simulink model "sysgenStreamedFFT"  (Simulink 7.4)
settings: Solver=VariableStepDiscrete  StartTime=0.0  StopTime=3000  RelTol=1e-3
values from neighbouring files (symbols this model uses):
  blue = blue(1:(min_x*min_y))    [makematrix.m]    (also in rgb.mat = [0 0 0 255 255 255 255 255 255 0 0 0 ... (256 elements, 256x)
  c = c(:)    [cellpipe_r13.m]    (also in cordic_sincos_script.m = xSignal; get_pipestr_r13.m = cellpipe_r13(pipestr))
  comp = [zeros(70,2) [zeros(2,66); comp; zeros(2,66)] zeros(70,2)]    [sysgenDWT_StopFcn.m]
undefined symbols (not defined in the file or in its folder): gcbh, xlBlockLoadCallback, xlipgetpartsetting
libraries: xbsIndex_r4 x117, dspxfrm3 x2, xbsCopyrightNotice_r4 x1
(part 1 of 3)
settings Model: Creator=douangp  LastModifiedBy=douangp
settings OptimizationCC: InitFltsAndDblsToZero=on
settings DebuggingCC: SaveWithParameterizedLinksMsg=none  SignalResolutionControl=TryResolveAllWithWarning  MultiTaskDSMMsg=warning  MultiTaskCondExecSysMsg=none
settings RTWCC: IncludeERTFirstTime=on
settings GRTTargetCC: TargetFcnLib=ansi_tfl_tmw.mat

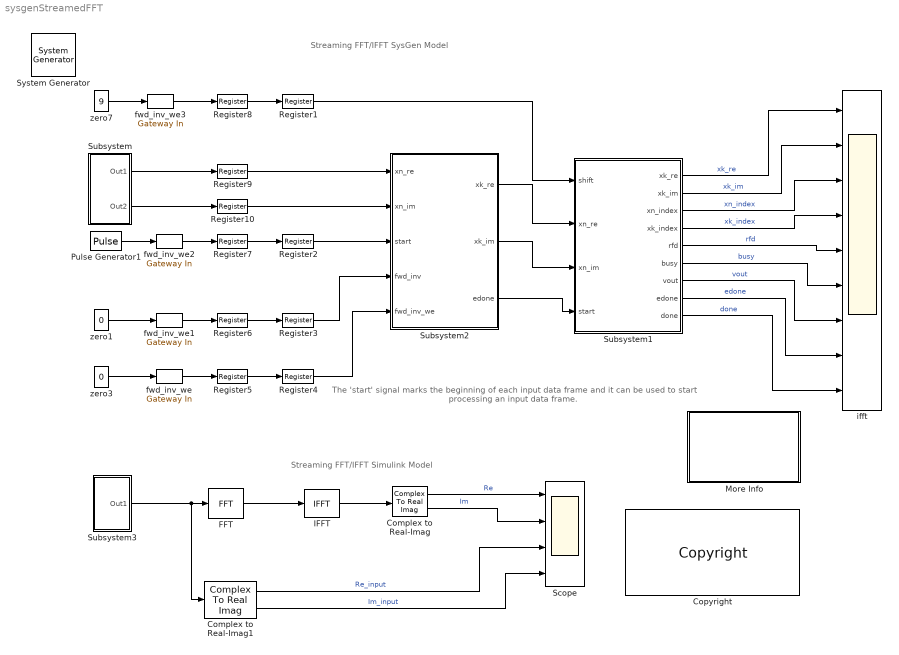
== system sysgenStreamedFFT ==
  note: The 'start' signal marks the beginning of each input data
      | frame and it can be used to start processing an input data frame.
  note: Streaming FFT/IFFT Simulink Model
  note: Streaming FFT/IFFT SysGen Model
  " System Generator" : xbsIndex_r4/ System Generator  Tag=genX  SystemSampleTime=-1  xilinxfamily=virtex6  part=xc6vlx240t  speed=-1  package=ff1156  synthesis_tool=XST  clock_wrapper=Clock Enables  directory=./timing  testbench=off  simulink_period=1  sysclk_period=5  dcm_input_clock_period=100  incr_netlist=off  trim_vbits=Everywhere in SubSystem  dbl_ovrd=According to Block Masks  core_generation=According to Block Masks  run_coregen=off  deprecated_control=off  eval_field=0  block_type=sysgen
      settings: block_version=9.1
  Complex to Real-Imag : ComplexToRealImag
  Complex to Real-Imag1 : ComplexToRealImag
  Copyright : xbsCopyrightNotice_r4/Copyright  copyrighttext="Copyright (c) 2010  by  Xilinx, Inc. All rights reserved.<br><br>This file contains proprietary, confidential information of Xilinx, Inc., is distributed under licensefrom Xilinx, Inc., and may be used, copied and/or disclosed only pursuant to the terms of a valid licenseagreement with Xilinx, Inc. Xilinx hereby grants you a license to use this file solely for design,simulation, implementation and creation of design files limited to Xilinx devices or technologies. Use with non-Xilinx devices or technologies is expressly prohibited and immediately terminates your license unless covered by a separate agreement.<br><br>Xilinx is providing this design, code, or information \"as-is\" solely for use in developing programs and solutions for Xilinx devices, with no obligation on the part of Xilinx to provide support. By providingthis design, code, or information as one possible implementation of this feature, application or standard,Xilinx is making no representation that this implementation is free from any claims of infringement. Youare responsible for obtaining any rights you may require for your implementation. Xilinx expressly disclaimsany warranty whatsoever with respect to the adequacy of the implementation, including but not limited to anywarranties or representations that this implementation is free from claims of infringement, implied warrantiesof merchantability or fitness for a particular purpose.<br><br>Xilinx products are not intended for use in life support appliances, devices, or systems. Use in such applications is expressly prohibited.<br><br>Any modifications that are made to the Source Code are done at the user's sole risk and will be unsupported.<br><br>This copyright and support notice must be retained as part of this text at all times. (c) Copyright 1995-2010 Xilinx, Inc. All rights reserved."  block_type=copyright
      settings: block_version=10.1.00
      settings: infoedit=|
      | Copyright(C) 2008 by  Xilinx, Inc. All rights reserved.<br>
      | <br>
      | This file contains proprietary, confidential information of Xilinx, Inc., is distributed under license
      | from Xilinx, Inc., and may be used, copied and/or disclosed only pursuant to the terms of a valid license
      | agreement with Xilinx, Inc. Xilinx hereby grants you a license to use this file solely for design,
      | simulation, implementation and creation of design files limited to Xilinx devices or technologies. Use
      | with non-Xilinx devices or technologies is expressly prohibited and immediately terminates your license
      | unless covered by a separate agreement.<br>
      | <br>
      | Xilinx is providing this design, code, or information "as-is" solely for use in developing programs and
      | solutions for Xilinx devices, with no obligation on the part of Xilinx to provide support. By providing
      | this design, code, or information as one possible implementation of this feature, application or standard,
      | Xilinx is making no representation that this implementation is free from any claims of infringement. You
      | are responsible for obtaining any rights you may require for your implementation. Xilinx expressly disclaims
      | any warranty whatsoever with respect to the adequacy of the implementation, including but not limited to any
      | warranties or representations that this implementation is free from claims of infringement, implied warranties
      | of merchantability or fitness for a particular purpose.<br>
      | <br>
      | Xilinx products are not intended for use in life support appliances, devices, or systems. Use in such
      | applications is expressly prohibited.<br>
      | <br>
      | Any modifications that are made to the Source Code are done at the user's sole risk and will be unsupported.<br>
      | <br>
      | This copyright and support notice must be retained as part of this text at all times.
      | (c) Copyright 1995-2008 Xilinx, Inc. All rights reserved.
  FFT : dspxfrm3/FFT  DialogController=dspDDGCreate  DialogControllerArgs=DataTag1  CompMethod=Table lookup  TableOpt=HYBRID  TableOptActive=Speed  BitRevOrder=off  InheritFFTLength=on  FFTLength=64  SkipNorm=off  roundingMode=Floor  overflowMode=off
  IFFT : dspxfrm3/IFFT  DialogController=dspDDGCreate  DialogControllerArgs=DataTag2  CompMethod=Table lookup  TableOpt=HYBRID  TableOptActive=Speed  BitRevOrder=off  cs_in=off  SkipNorm=on  InheritFFTLength=on  FFTLength=64  mode=Complex  outSamplingMode=Frame based  roundingMode=Floor  overflowMode=off
  More Info : Subsystem
      mask Display: disp('Double click\n for\n more information.')
  Pulse Generator1 : DiscretePulseGenerator  Amplitude=1  Period=10000  PulseWidth=9999  PhaseDelay=2  SampleTime=1
  Register{1..10} (10 alike) : xbsIndex_r4/Register  init=0  rst=off  en=off  dbl_ovrd=off  block_type=register
      settings: block_version=9.1
  Scope : Scope  NumInputPorts=4
      settings: TimeRange=100  YMin=5.55112e-017~-1~5.55112e-017~-1  YMax=1~1~1~1  SaveName=ScopeData3
  Subsystem : Subsystem
  Subsystem1 : Subsystem
  Subsystem2 : Subsystem
  Subsystem3 : Subsystem
  fwd_inv_we : xbsIndex_r4/Gateway In  arith_type=Boolean  n_bits=16  bin_pt=0  quantization=Truncate  overflow=Wrap  period=1  dbl_ovrd=off  timing_constraint=None  locs_specified=off  LOCs={}  hdl_port=on  block_type=gatewayin
      settings: infoedit="Gateway in block.  Converts inputs of type Simulink integer, double and fixed point to  Xilinx fixed point type.<P><P>Hardware notes:  In hardware these blocks become top level input ports."  xl_area=[0, 0, 0, 0, 0, 0, 0]  block_version=8.2.02
  fwd_inv_we1 : xbsIndex_r4/Gateway In  arith_type=Boolean  n_bits=16  bin_pt=0  quantization=Truncate  overflow=Wrap  period=1  dbl_ovrd=off  timing_constraint=None  locs_specified=off  LOCs={}  hdl_port=on  block_type=gatewayin
      settings: infoedit="Gateway in block.  Converts inputs of type Simulink integer, double and fixed point to  Xilinx fixed point type.<P><P>Hardware notes:  In hardware these blocks become top level input ports."  xl_area=[0, 0, 0, 0, 0, 0, 0]  block_version=8.2.02
  fwd_inv_we2 : xbsIndex_r4/Gateway In  arith_type=Boolean  n_bits=16  bin_pt=0  quantization=Truncate  overflow=Wrap  period=1  dbl_ovrd=off  timing_constraint=None  locs_specified=off  LOCs={}  hdl_port=on  block_type=gatewayin
      settings: infoedit="Gateway in block.  Converts inputs of type Simulink integer, double and fixed point to  Xilinx fixed point type.<P><P>Hardware notes:  In hardware these blocks become top level input ports."  xl_area=[0, 0, 0, 0, 0, 0, 0]  block_version=8.2.02
  fwd_inv_we3 : xbsIndex_r4/Gateway In  arith_type=Unsigned  n_bits=4  bin_pt=0  quantization=Truncate  overflow=Wrap  period=1  dbl_ovrd=off  timing_constraint=None  locs_specified=off  LOCs={}  hdl_port=on  block_type=gatewayin
      settings: infoedit="Gateway in block.  Converts inputs of type Simulink integer, double and fixed point to  Xilinx fixed point type.<P><P>Hardware notes:  In hardware these blocks become top level input ports."  xl_area=[0, 0, 0, 0, 0, 0, 0]  block_version=8.2.02
  ifft : Scope  NumInputPorts=9
      settings: TimeRange=1000  YMin=-0.15~-0.15~0~0~0.95~0.95~0~0~0  YMax=0.15~0.15~300~300~1.05~1.05~1~1~1
  zero1 : Constant  Value=0  OutDataType=sfix(16)  OutScaling=2^0
  zero3 : Constant  Value=0  OutDataType=sfix(16)  OutScaling=2^0
  zero7 : Constant  Value=9  OutDataType=sfix(16)  OutScaling=2^0
  wires:
  Register10/1 -> Subsystem2/2(xn_im)
  Register4/1 -> Subsystem2/5(fwd_inv_we)
  fwd_inv_we/1 -> Register5/1
  zero3/1 -> fwd_inv_we/1
  Subsystem1/1(xk_re) -> ifft/1  "xk_re"
  Subsystem1/2(xk_im) -> ifft/2  "xk_im"
  Subsystem1/3(xn_index) -> ifft/3  "xn_index"
  Subsystem1/4(xk_index) -> ifft/4  "xk_index"
  Subsystem1/5(rfd) -> ifft/5  "rfd"
  Subsystem1/6(busy) -> ifft/6  "busy"
  Subsystem1/7(vout) -> ifft/7  "vout"
  Subsystem1/8(edone) -> ifft/8  "edone"
  Subsystem1/9(done) -> ifft/9  "done"
  Subsystem/2(Out2) -> Register10/1
  Subsystem/1(Out1) -> Register9/1
  Register5/1 -> Register4/1
  FFT/1 -> IFFT/1
  IFFT/1 -> Complex to Real-Imag/1
  Complex to Real-Imag/1 -> Scope/1  "Re"
  Complex to Real-Imag/2 -> Scope/2  "Im"
  Complex to Real-Imag1/2 -> Scope/4  "Im_input"
  Complex to Real-Imag1/1 -> Scope/3  "Re_input"
  Register9/1 -> Subsystem2/1(xn_re)
  Subsystem2/1(xk_re) -> Subsystem1/2(xn_re)
  Subsystem2/2(xk_im) -> Subsystem1/3(xn_im)
  Subsystem2/3(edone) -> Subsystem1/4(start)
  Subsystem3/1(Out1) -> FFT/1, Complex to Real-Imag1/1
  fwd_inv_we3/1 -> Register8/1
  zero7/1 -> fwd_inv_we3/1
  Register1/1 -> Subsystem1/1(shift)
  fwd_inv_we1/1 -> Register6/1
  Register6/1 -> Register3/1
  Register3/1 -> Subsystem2/4(fwd_inv)
  zero1/1 -> fwd_inv_we1/1
  fwd_inv_we2/1 -> Register7/1
  Register7/1 -> Register2/1
  Register2/1 -> Subsystem2/3(start)
  Register8/1 -> Register1/1
  Pulse Generator1/1 -> fwd_inv_we2/1

== system sysgenStreamedFFT/More Info ==
  note: This design demonstrates how the Xilinx FFT block can be used in a data stream with identical input and output rates.
      | In addition, the demo also shows how to incorporate DDS Compiler blocks and complex multipliers as a subsystem to this model.
      | Both Sine and Cosine output signals are used as inputs into the complex multipliers, realized and verified using Simulink, fixed-point simulation.
      | A Simulink model is provided for your reference only.
      |
      | Using SysGen and ISE 10.1, the following operating frequency is obtained for these two target devices:
      | -  Virtex-5 xc5vsx50t-1ff1136:  3.236 ns with 5 levels of logic
      | -  Spartan-3A DSP xc3sd3400a-4fg676: 5.655 ns with 7 levels of logic
  note: Streaming FFT/IFFT Demonstration

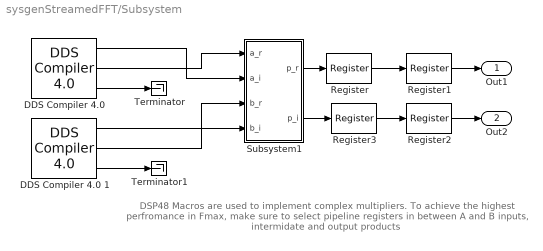
== system sysgenStreamedFFT/Subsystem ==
  note: DSP48 Macros are used to implement complex multipliers. To achieve
      | the highest perfromance in Fmax, make sure to select pipeline registers in between
      | A and B inputs, intermidate and output products
  "DDS Compiler 4.0 " : xbsIndex_r4/DDS Compiler 4.0   partspresent=Phase_Generator_and_SIN_COS_LUT  dds_clock_rate=100  channels=1  parameter_entry=System_Parameters  spurious_free_dynamic_range=36  frequency_resolution=0.4  noise_shaping=None  phase_width=28  output_width=6  output_selection=Sine_and_Cosine  negative_sine=off  negative_cosine=off  amplitude_mode=Full_Range  memory_type=Auto  optimization_goal=Auto  dsp48_use=Minimal  latency_configuration=Auto  latency=2  has_phase_out=on  sclr_pin=off  clock_enable=off  rfd=off  rdy=off  channel_pin=off  explicit_period=off  period=1  phase_increment=Fixed  output_frequency1=1  output_frequency2=0  output_frequency3=0  output_frequency4=0  output_frequency5=0  output_frequency6=0  output_frequency7=0  output_frequency8=0  output_frequency9=0  output_frequency10=0  output_frequency11=0  output_frequency12=0  output_frequency13=0  output_frequency14=0  output_frequency15=0  output_frequency16=0  pinc1='0'  pinc2='0'  pinc3='0'  pinc4='0'  pinc5='0'  pinc6='0'  pinc7='0'  pinc8='0'  pinc9='0'  pinc10='0'  pinc11='0'  pinc12='0'  pinc13='0'  pinc14='0'  pinc15='0'  pinc16='0'  phase_offset=None  phase_offset_angles1=0  phase_offset_angles2=0  phase_offset_angles3=0  phase_offset_angles4=0  phase_offset_angles5=0  phase_offset_angles6=0  phase_offset_angles7=0  phase_offset_angles8=0  phase_offset_angles9=0  phase_offset_angles10=0  phase_offset_angles11=0  phase_offset_angles12=0  phase_offset_angles13=0  phase_offset_angles14=0  phase_offset_angles15=0  phase_offset_angles16=0  poff1='0'  poff2='0'  poff3='0'  poff4='0'  poff5='0'  poff6='0'  poff7='0'  poff8='0'  poff9='0'  poff10='0'  poff11='0'  poff12='0'  poff13='0'  poff14='0'  poff15='0'  poff16='0'  por_mode=false  gui_behaviour=Sysgen  ip_name=DDS Compiler  ip_version=4.0  dsptool_ready=true  wrapper_available=true  port_translation_map={ 'ce' => 'en', 'sclr' => 'rst' }  ipcore_xco_need_fpga_part=true  ipcore_fpga_part=xlipgetpartsetting(gcb, {'virtex4', 'xc4vsx35', '-10', 'ff668'})  ipcore_usecache=true  ipcore_useipmodelcache=true  ipcore_verbose=false  block_type=dds_compiler_v4_0
      settings: block_version=11.3
  DDS Compiler 4.0 1 : xbsIndex_r4/DDS Compiler 4.0   partspresent=Phase_Generator_and_SIN_COS_LUT  dds_clock_rate=100  channels=1  parameter_entry=System_Parameters  spurious_free_dynamic_range=36  frequency_resolution=0.4  noise_shaping=None  phase_width=28  output_width=6  output_selection=Sine_and_Cosine  negative_sine=off  negative_cosine=off  amplitude_mode=Full_Range  memory_type=Auto  optimization_goal=Auto  dsp48_use=Minimal  latency_configuration=Auto  latency=2  has_phase_out=on  sclr_pin=off  clock_enable=off  rfd=off  rdy=off  channel_pin=off  explicit_period=off  period=1  phase_increment=Fixed  output_frequency1=1  output_frequency2=0  output_frequency3=0  output_frequency4=0  output_frequency5=0  output_frequency6=0  output_frequency7=0  output_frequency8=0  output_frequency9=0  output_frequency10=0  output_frequency11=0  output_frequency12=0  output_frequency13=0  output_frequency14=0  output_frequency15=0  output_frequency16=0  pinc1='0'  pinc2='0'  pinc3='0'  pinc4='0'  pinc5='0'  pinc6='0'  pinc7='0'  pinc8='0'  pinc9='0'  pinc10='0'  pinc11='0'  pinc12='0'  pinc13='0'  pinc14='0'  pinc15='0'  pinc16='0'  phase_offset=None  phase_offset_angles1=0  phase_offset_angles2=0  phase_offset_angles3=0  phase_offset_angles4=0  phase_offset_angles5=0  phase_offset_angles6=0  phase_offset_angles7=0  phase_offset_angles8=0  phase_offset_angles9=0  phase_offset_angles10=0  phase_offset_angles11=0  phase_offset_angles12=0  phase_offset_angles13=0  phase_offset_angles14=0  phase_offset_angles15=0  phase_offset_angles16=0  poff1='0'  poff2='0'  poff3='0'  poff4='0'  poff5='0'  poff6='0'  poff7='0'  poff8='0'  poff9='0'  poff10='0'  poff11='0'  poff12='0'  poff13='0'  poff14='0'  poff15='0'  poff16='0'  por_mode=false  gui_behaviour=Sysgen  ip_name=DDS Compiler  ip_version=4.0  dsptool_ready=true  wrapper_available=true  port_translation_map={ 'ce' => 'en', 'sclr' => 'rst' }  ipcore_xco_need_fpga_part=true  ipcore_fpga_part=xlipgetpartsetting(gcb, {'virtex4', 'xc4vsx35', '-10', 'ff668'})  ipcore_usecache=true  ipcore_useipmodelcache=true  ipcore_verbose=false  block_type=dds_compiler_v4_0
      settings: block_version=11.3
  Register{,1..3} (4 alike) : xbsIndex_r4/Register  init=0  rst=off  en=off  dbl_ovrd=off  block_type=register
      settings: block_version=9.1
  Subsystem1 : Subsystem
  Terminator : Terminator
  Terminator1 : Terminator
  Out1 : Outport  OutDataType=sfix(16)  OutScaling=2^0
  Out2 : Outport  Port=2  OutDataType=sfix(16)  OutScaling=2^0
  wires:
  Subsystem1/1(p_r) -> Register/1
  Subsystem1/2(p_i) -> Register3/1
  Register/1 -> Register1/1
  Register3/1 -> Register2/1
  Register1/1 -> Out1/1
  Register2/1 -> Out2/1
  "DDS Compiler 4.0 "/1 -> Subsystem1/2(a_i)
  "DDS Compiler 4.0 "/2 -> Subsystem1/1(a_r)
  DDS Compiler 4.0 1/1 -> Subsystem1/4(b_i)
  DDS Compiler 4.0 1/2 -> Subsystem1/3(b_r)
  "DDS Compiler 4.0 "/3 -> Terminator/1
  DDS Compiler 4.0 1/3 -> Terminator1/1

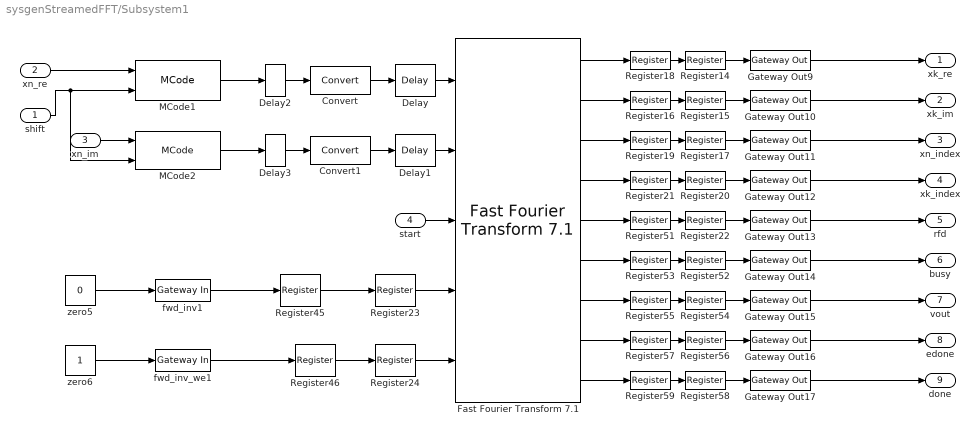
== system sysgenStreamedFFT/Subsystem1 ==
  shift : Inport  OutDataType=sfix(16)  OutScaling=2^0
  xn_re : Inport  Port=2  OutDataType=sfix(16)  OutScaling=2^0
  xn_im : Inport  Port=3  OutDataType=sfix(16)  OutScaling=2^0
  start : Inport  Port=4  OutDataType=sfix(16)  OutScaling=2^0
  Convert : xbsIndex_r4/Convert  arith_type="Signed  (2's comp)"  n_bits=16  bin_pt=15  quantization=Truncate  overflow=Wrap  en=off  latency=1  dbl_ovrd=off  pipeline=off  block_type=convert
      settings: block_version=9.1
  Convert1 : xbsIndex_r4/Convert  arith_type="Signed  (2's comp)"  n_bits=16  bin_pt=15  quantization=Truncate  overflow=Wrap  en=off  latency=1  dbl_ovrd=off  pipeline=off  block_type=convert
      settings: block_version=9.1
  Delay{,1..3} (4 alike) : xbsIndex_r4/Delay  en=off  latency=1  dbl_ovrd=off  reg_retiming=off  block_type=delay
      settings: block_version=9.1
  "Fast Fourier Transform 7.1 " : xbsIndex_r4/Fast Fourier Transform 7.1   transform_length=256  implementation_options=pipelined_streaming_io  target_clock_frequency=250  target_data_throughput=50  run_time_configurable_transform_length=off  phase_factor_width=16  scaling_options=unscaled  rounding_modes=convergent_rounding  output_ordering=natural_order  cyclic_prefix_insertion=off  ce=off  sclr=off  ovflo=off  input_data_offset=no_offset  memory_options_data=block_ram  memory_options_phase_factors=block_ram  number_of_stages_using_block_ram_for_data_and_phase_factors=3  memory_options_reorder=block_ram  memory_options_hybrid=off  complex_mult_type=use_mults_resources  butterfly_type=use_luts  channels=1  input_ordering=natural_order  input_width=16  simulation_type=external_xfix  simulation_model=fftv71_CModel:fftv71_cmodel  ip_name=Fast Fourier Transform  ip_version=7.1  dsptool_ready=true  wrapper_available=true  port_translation_map={ 'ce' => 'en', 'sclr' => 'rst' }  ipcore_fpga_part=xlipgetpartsetting(gcb, {'virtex4', 'xc4vsx35', '-10', 'ff668'})  block_type=xfft_v7_1
      settings: block_version=12.1
  Gateway Out{9..17} (9 alike) : xbsIndex_r4/Gateway Out  hdl_port=on  timing_constraint=None  locs_specified=off  LOCs={}  block_type=gatewayout
      settings: infoedit="Gateway out block.  Converts Xilinx fixed point inputs into ouputs of type Simulink integer, double, or fixed point.<P><P>Hardware notes:  In hardware these blocks become top level output ports or are discarded, depending on how they are configured."  block_version=9.1
  MCode1 : xbsIndex_r4/MCode  mfname=x_shift  explicit_period=off  period=1  inputsTable={'boundInpExpr'=>['',''],'inputs'=>['din','shift']}  outputsTable={'outputs'=>['dout'],'suppressOut'=>['off']}  dbl_ovrd=off  enable_stdout=off  enable_debug=off  suppress_output=off  defparams={}  hide_port_list={}  block_type=mcode
      settings: xl_area=[0, 0, 0, 0, 0, 0, 0]  block_version=8.1
  MCode2 : xbsIndex_r4/MCode  mfname=x_shift  explicit_period=off  period=1  inputsTable={'boundInpExpr'=>['',''],'inputs'=>['din','shift']}  outputsTable={'outputs'=>['dout'],'suppressOut'=>['off']}  dbl_ovrd=off  enable_stdout=off  enable_debug=off  suppress_output=off  defparams={}  hide_port_list={}  block_type=mcode
      settings: xl_area=[0, 0, 0, 0, 0, 0, 0]  block_version=8.1
  Register{14..24,45..46,51..59} (22 alike) : xbsIndex_r4/Register  init=0  rst=off  en=off  dbl_ovrd=off  block_type=register
      settings: block_version=9.1
  fwd_inv1 : xbsIndex_r4/Gateway In  arith_type=Boolean  n_bits=16  bin_pt=0  quantization=Truncate  overflow=Wrap  period=1  dbl_ovrd=off  timing_constraint=None  locs_specified=off  LOCs={}  hdl_port=on  block_type=gatewayin
      settings: infoedit="Gateway in block.  Converts inputs of type Simulink integer, double and fixed point to  Xilinx fixed point type.<P><P>Hardware notes:  In hardware these blocks become top level input ports."  xl_area=[0, 0, 0, 0, 0, 0, 0]  block_version=8.2.02
  fwd_inv_we1 : xbsIndex_r4/Gateway In  arith_type=Boolean  n_bits=16  bin_pt=0  quantization=Truncate  overflow=Wrap  period=1  dbl_ovrd=off  timing_constraint=None  locs_specified=off  LOCs={}  hdl_port=on  block_type=gatewayin
      settings: infoedit="Gateway in block.  Converts inputs of type Simulink integer, double and fixed point to  Xilinx fixed point type.<P><P>Hardware notes:  In hardware these blocks become top level input ports."  xl_area=[0, 0, 0, 0, 0, 0, 0]  block_version=8.2.02
  zero5 : Constant  Value=0  OutDataType=sfix(16)  OutScaling=2^0
  zero6 : Constant  OutDataType=sfix(16)  OutScaling=2^0
  xk_re : Outport  OutDataType=sfix(16)  OutScaling=2^0
  xk_im : Outport  Port=2  OutDataType=sfix(16)  OutScaling=2^0
  xn_index : Outport  Port=3  OutDataType=sfix(16)  OutScaling=2^0
  xk_index : Outport  Port=4  OutDataType=sfix(16)  OutScaling=2^0
  rfd : Outport  Port=5  OutDataType=sfix(16)  OutScaling=2^0
  busy : Outport  Port=6  OutDataType=sfix(16)  OutScaling=2^0
  vout : Outport  Port=7  OutDataType=sfix(16)  OutScaling=2^0
  edone : Outport  Port=8  OutDataType=sfix(16)  OutScaling=2^0
  done : Outport  Port=9  OutDataType=sfix(16)  OutScaling=2^0
  wires:
  "Fast Fourier Transform 7.1 "/1 -> Register18/1
  Register18/1 -> Register14/1
  "Fast Fourier Transform 7.1 "/2 -> Register16/1
  Register16/1 -> Register15/1
  "Fast Fourier Transform 7.1 "/3 -> Register19/1
  Register19/1 -> Register17/1
  "Fast Fourier Transform 7.1 "/4 -> Register21/1
  Register21/1 -> Register20/1
  Register51/1 -> Register22/1
  Register53/1 -> Register52/1
  Register55/1 -> Register54/1
  Register57/1 -> Register56/1
  Register59/1 -> Register58/1
  "Fast Fourier Transform 7.1 "/5 -> Register51/1
  "Fast Fourier Transform 7.1 "/6 -> Register53/1
  "Fast Fourier Transform 7.1 "/7 -> Register55/1
  "Fast Fourier Transform 7.1 "/8 -> Register57/1
  "Fast Fourier Transform 7.1 "/9 -> Register59/1
  fwd_inv1/1 -> Register45/1
  fwd_inv_we1/1 -> Register46/1
  zero5/1 -> fwd_inv1/1
  zero6/1 -> fwd_inv_we1/1
  Register23/1 -> "Fast Fourier Transform 7.1 "/4
  Convert/1 -> Delay/1
  Convert1/1 -> Delay1/1
  Delay/1 -> "Fast Fourier Transform 7.1 "/1
  Delay1/1 -> "Fast Fourier Transform 7.1 "/2
  Delay2/1 -> Convert/1
  Delay3/1 -> Convert1/1
  Register24/1 -> "Fast Fourier Transform 7.1 "/5
  Register45/1 -> Register23/1
  Register46/1 -> Register24/1
  Register14/1 -> Gateway Out9/1
  Register15/1 -> Gateway Out10/1
  Register17/1 -> Gateway Out11/1
  Register20/1 -> Gateway Out12/1
  Register22/1 -> Gateway Out13/1
  Register52/1 -> Gateway Out14/1
  Register54/1 -> Gateway Out15/1
  Register56/1 -> Gateway Out16/1
  Register58/1 -> Gateway Out17/1
  xn_re/1 -> MCode1/1
  xn_im/1 -> MCode2/1
  start/1 -> "Fast Fourier Transform 7.1 "/3
  Gateway Out9/1 -> xk_re/1
  Gateway Out10/1 -> xk_im/1
  Gateway Out11/1 -> xn_index/1
  Gateway Out12/1 -> xk_index/1
  Gateway Out13/1 -> rfd/1
  Gateway Out14/1 -> busy/1
  Gateway Out15/1 -> vout/1
  Gateway Out16/1 -> edone/1
  Gateway Out17/1 -> done/1
  MCode1/1 -> Delay2/1
  MCode2/1 -> Delay3/1
  shift/1 -> MCode2/2, MCode1/2

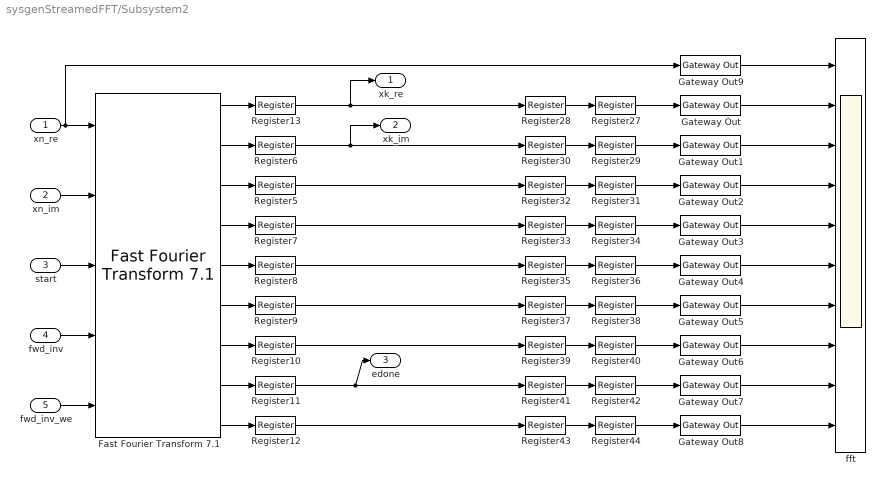
== system sysgenStreamedFFT/Subsystem2 ==
  xn_re : Inport  OutDataType=sfix(16)  OutScaling=2^0
  xn_im : Inport  Port=2  OutDataType=sfix(16)  OutScaling=2^0
  start : Inport  Port=3  OutDataType=sfix(16)  OutScaling=2^0
  fwd_inv : Inport  Port=4  OutDataType=sfix(16)  OutScaling=2^0
  fwd_inv_we : Inport  Port=5  OutDataType=sfix(16)  OutScaling=2^0
  "Fast Fourier Transform 7.1 " : xbsIndex_r4/Fast Fourier Transform 7.1   transform_length=256  implementation_options=pipelined_streaming_io  target_clock_frequency=250  target_data_throughput=50  run_time_configurable_transform_length=off  phase_factor_width=16  scaling_options=unscaled  rounding_modes=convergent_rounding  output_ordering=natural_order  cyclic_prefix_insertion=off  ce=off  sclr=off  ovflo=off  input_data_offset=no_offset  memory_options_data=block_ram  memory_options_phase_factors=block_ram  number_of_stages_using_block_ram_for_data_and_phase_factors=3  memory_options_reorder=block_ram  memory_options_hybrid=off  complex_mult_type=use_mults_resources  butterfly_type=use_luts  channels=1  input_ordering=natural_order  input_width=16  simulation_type=external_xfix  simulation_model=fftv71_CModel:fftv71_cmodel  ip_name=Fast Fourier Transform  ip_version=7.1  dsptool_ready=true  wrapper_available=true  port_translation_map={ 'ce' => 'en', 'sclr' => 'rst' }  ipcore_fpga_part=xlipgetpartsetting(gcb, {'virtex4', 'xc4vsx35', '-10', 'ff668'})  block_type=xfft_v7_1
      settings: block_version=12.1
  Gateway Out{,1..8} (9 alike) : xbsIndex_r4/Gateway Out  hdl_port=on  timing_constraint=None  locs_specified=off  LOCs={}  block_type=gatewayout
      settings: infoedit="Gateway out block.  Converts Xilinx fixed point inputs into ouputs of type Simulink integer, double, or fixed point.<P><P>Hardware notes:  In hardware these blocks become top level output ports or are discarded, depending on how they are configured."  block_version=9.1
  Gateway Out9 : xbsIndex_r4/Gateway Out  hdl_port=off  timing_constraint=None  locs_specified=off  LOCs={}  block_type=gatewayout
      settings: infoedit="Gateway out block.  Converts Xilinx fixed point inputs into ouputs of type Simulink integer, double, or fixed point.<br><br>Hardware notes:  In hardware these blocks become top level output ports or are discarded, depending on how they are configured."  block_version=9.1
  Register{5..13,27..44} (27 alike) : xbsIndex_r4/Register  init=0  rst=off  en=off  dbl_ovrd=off  block_type=register
      settings: block_version=9.1
  fft : Scope  NumInputPorts=10
      settings: TimeRange=1200  YMin=-0.002~-0.1~-0.5~0~0~0~0~0~0~0  YMax=0.002~0.1~0.5~400~400~1~1~1~1~1
  xk_re : Outport  OutDataType=sfix(16)  OutScaling=2^0
  xk_im : Outport  Port=2  OutDataType=sfix(16)  OutScaling=2^0
  edone : Outport  Port=3  OutDataType=sfix(16)  OutScaling=2^0
  wires:
  xn_re/1 -> Gateway Out9/1, "Fast Fourier Transform 7.1 "/1
  Gateway Out/1 -> fft/2
  Gateway Out1/1 -> fft/3
  Gateway Out2/1 -> fft/4
  Gateway Out3/1 -> fft/5
  Gateway Out4/1 -> fft/6
  Gateway Out5/1 -> fft/7
  Gateway Out6/1 -> fft/8
  Gateway Out7/1 -> fft/9
  Gateway Out8/1 -> fft/10
  Register27/1 -> Gateway Out/1
  Register29/1 -> Gateway Out1/1
  Register31/1 -> Gateway Out2/1
  Register34/1 -> Gateway Out3/1
  Register36/1 -> Gateway Out4/1
  Register38/1 -> Gateway Out5/1
  Register40/1 -> Gateway Out6/1
  Register42/1 -> Gateway Out7/1
  Register44/1 -> Gateway Out8/1
  "Fast Fourier Transform 7.1 "/9 -> Register12/1
  "Fast Fourier Transform 7.1 "/8 -> Register11/1
  "Fast Fourier Transform 7.1 "/7 -> Register10/1
  "Fast Fourier Transform 7.1 "/6 -> Register9/1
  "Fast Fourier Transform 7.1 "/5 -> Register8/1
  "Fast Fourier Transform 7.1 "/4 -> Register7/1
  "Fast Fourier Transform 7.1 "/3 -> Register5/1
  "Fast Fourier Transform 7.1 "/2 -> Register6/1
  "Fast Fourier Transform 7.1 "/1 -> Register13/1
  Register13/1 -> Register28/1, xk_re/1
  Register6/1 -> Register30/1, xk_im/1
  Register5/1 -> Register32/1
  Register7/1 -> Register33/1
  Register8/1 -> Register35/1
  Register9/1 -> Register37/1
  Register10/1 -> Register39/1
  Register11/1 -> Register41/1, edone/1
  Register12/1 -> Register43/1
  Register28/1 -> Register27/1
  Register30/1 -> Register29/1
  Register32/1 -> Register31/1
  Register33/1 -> Register34/1
  Register35/1 -> Register36/1
  Register37/1 -> Register38/1
  Register39/1 -> Register40/1
  Register41/1 -> Register42/1
  Register43/1 -> Register44/1
  xn_im/1 -> "Fast Fourier Transform 7.1 "/2
  start/1 -> "Fast Fourier Transform 7.1 "/3
  fwd_inv/1 -> "Fast Fourier Transform 7.1 "/4
  fwd_inv_we/1 -> "Fast Fourier Transform 7.1 "/5
  Gateway Out9/1 -> fft/1

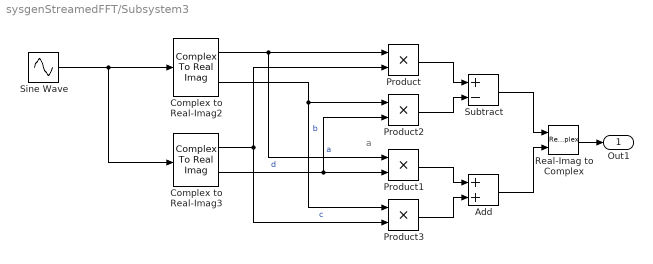
== system sysgenStreamedFFT/Subsystem3 ==
  note: a
  Add : Sum  OutDataType=sfix(16)  OutScaling=2^-10
  Complex to Real-Imag2 : ComplexToRealImag
  Complex to Real-Imag3 : ComplexToRealImag
  Product{,1..3} (4 alike) : Product  OutDataType=sfix(16)  OutScaling=2^0  RndMeth=Zero
  Real-Imag to Complex : RealImagToComplex
  Sine Wave : Sin  Amplitude=1  Bias=0  Frequency=1  Phase=0  Samples=10  SampleTime=1/100  Offset=0
  Subtract : Sum  Inputs=+-  OutDataType=sfix(16)  OutScaling=2^-10
  Out1 : Outport  OutDataType=sfix(16)  OutScaling=2^0
  wires:
  Complex to Real-Imag2/1 -> Product/1, Product1/1  "a"
  Complex to Real-Imag2/2 -> Product2/1, Product3/1  "b"
  Complex to Real-Imag3/1 -> Product3/2, Product/2  "c"
  Complex to Real-Imag3/2 -> Product1/2, Product2/2  "d"
  Product/1 -> Subtract/1
  Product2/1 -> Subtract/2
  Product1/1 -> Add/1
  Product3/1 -> Add/2
  Subtract/1 -> Real-Imag to Complex/1
  Add/1 -> Real-Imag to Complex/2
  Sine Wave/1 -> Complex to Real-Imag2/1, Complex to Real-Imag3/1
  Real-Imag to Complex/1 -> Out1/1
